simulink model "LEGO_PendulumOnCart"  (R2013b)
settings: Solver=ode3  SolverMode=SingleTasking  StartTime=0.0  StopTime=13  FixedStep=ts1  RelTol=1e-3
PostLoadFcn:
  | LEGO_PendulumOnCart_plant;
  | LEGO_PendulumOnCart_controller;
  | LEGO_PendulumOnCart_simulation;
InitFcn:
  | LEGO_PendulumOnCart_plant;
  | LEGO_PendulumOnCart_controller;
  | LEGO_PendulumOnCart_simulation;
values from neighbouring files (symbols this model uses):
  a_b = 0.8    [LEGO_PendulumOnCart_controller.m]    (also in matlab.mat)
  a_d = 0.8    [LEGO_PendulumOnCart_controller.m]    (also in matlab.mat)
  ANGLE_OFFSET = 93    [LEGO_PendulumOnCart_controller.m]    (also in matlab.mat = 48)
  cm2phi = 2    [LEGO_PendulumOnCart_controller.m]    (also in matlab.mat = 1)
  k_cp = 0.5    [matlab.mat]
  k_gv = w_n^2/(212.4*k_v)    (= 1.61490625454)    [LEGO_PendulumOnCart_controller.m]    (also in matlab.mat)
  k_v = (w_n^2-2826)/212.4    (= 21.6375823917)    [LEGO_PendulumOnCart_controller.m]    (also in matlab.mat)
  k_z = -2*w_n1    [LEGO_PendulumOnCart_controller.m]    (also in matlab.mat = -15.1928775883)
  l = 0.17    [LEGO_PendulumOnCart_controller.m]    (also in LEGO_PendulumOnCart_plant.m; matlab.mat)
  R = 0.025    [LEGO_PendulumOnCart_plant.m]    (also in matlab.mat)
  ts1 = 0.004    [LEGO Servo Motor experiments.mat]    (also in LEGO_PendulumOnCart_controller.m; matlab.mat)
undefined symbols (not defined in the file or in its folder): Normalized, sigbuilder_block
libraries: legonxtlib x10, simulink x3
CloseFcn:
  | LEGO_PendulumOnCart_closemodel;
Description:
  | This is an Implementation of Pendulum on a cart system using LEGO Mindstorms NXT Kit.
settings Model: ExtModeTrigDuration=2  Creator=Alphonso Monk  LastModifiedBy=Alphonso Monk
settings OptimizationCC: OptimizeModelRefInitCode=on  LifeSpan=1
settings DebuggingCC: SolverPrmCheckMsg=none
settings HardwareCC: ProdLargestAtomicInteger=Long  ProdLargestAtomicFloat=Float  ProdEndianess=LittleEndian  ProdHWDeviceType=ARM Compatible->ARM 7
settings SFSimCC: SimParseCustomCode=off
settings RTWCC: SystemTargetFile=realtime.tlc  GenerateMakefile=off  TemplateMakefile=realtime.tmf  Description=Run on Target Hardware  RTWVerbose=off  ProcessScript=realtime_make_rtw_hook
settings CodeAppCC: InternalIdentifier=Classic
settings STFCustomTargetCC: TargetLibSuffix=.a  GenerateSampleERTMain=on  ERTCustomFileBanners=on  SupportNonInlinedSFcns=off  SupportVariableSizeSignals=on  MATLABClassNameForMDSCustomization=Simulink.SoftwareTarget.ERTCustomization  GRTInterface=off  SystemTargetFile=realtime.tlc
settings ERTTargetCC: CodeReplacementLibrary=ANSI_C  GenerateSampleERTMain=on  ParMdlRefBuildCompliant=off  CompOptLevelCompliant=off  ConcurrentExecutionCompliant=off  CombineOutputUpdateFcns=off  ERTFirstTimeCompliant=off  SupportContinuousTime=on  SupportVariableSizeSignals=on  ModelStepFunctionPrototypeControlCompliant=off  CPPClassGenCompliant=off  ExtMode=on  ExtModeTransport=2  ExtModeMexFile=ext_serial_win32_comm_no_acks_rtt  ExtModeMexArgs=0 3 9600 30  InlinedParameterPlacement=NonHierarchical  ERTSrcFileBannerTemplate=realtime_code_template.cgt  ERTHdrFileBannerTemplate=realtime_code_template.cgt  ERTDataSrcFileTemplate=realtime_code_template.cgt  ERTDataHdrFileTemplate=realtime_code_template.cgt  ERTCustomFileTemplate=realtime_file_process.tlc

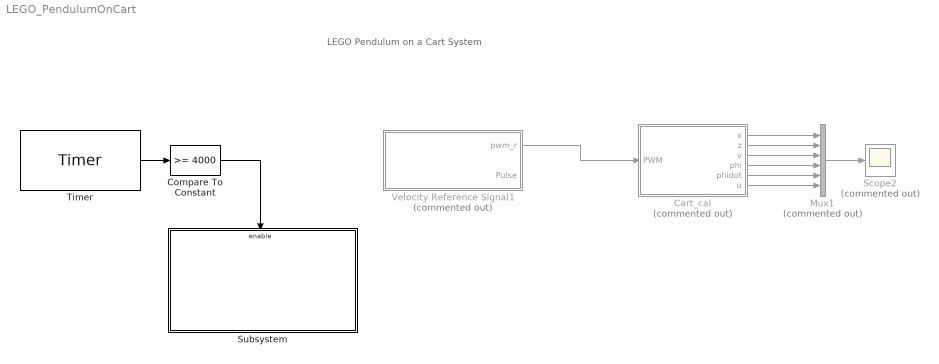
== system LEGO_PendulumOnCart ==
  note: LEGO Pendulum on a Cart System
  Cart_cal : Subsystem  Commented=on
  Compare To Constant : simulink/Logic and Bit Operations/Compare To Constant  relop=>=  const=4000  OutDataTypeStr=boolean
  Mux1 : Mux  Commented=on  Inputs=6
  Scope2 : Scope  Commented=on
      settings: YMin=-25  YMax=50  SaveName=PendulumOnCart_scope2
  Subsystem : Subsystem
  Timer : legonxtlib/Timer  sampleTime=0.1
  Velocity Reference Signal1 : Subsystem  Tag=STV Subsys  Commented=on  LoadFcn=sigbuilder_block('load');  StartFcn=sigbuilder_block('start');  StopFcn=sigbuilder_block('stop');  ClipboardFcn=sigbuilder_block('clipboard');  mask(Sigbuilder block){}
      mask help: Simulink:masks:SigbuilderBlock_MD
      mask init:
      | if ~strcmp(get_param(bdroot(gcbh),'SimulationStatus'),'stopped') tuvar = sigbuilder_block('maskInit'); end
      settings: CopyFcn=sigbuilder_block('copy');  DeleteFcn=sigbuilder_block('delete');  ModelCloseFcn=sigbuilder_block('modelClose');  PreSaveFcn=sigbuilder_block('preSave');  PauseFcn=sigbuilder_block('pause');  ContinueFcn=sigbuilder_block('continue');  NameChangeFcn=sigbuilder_block('namechange');  OpenFcn=sigbuilder_block('open',[437.25 118.5 550.5 394.5 ]);  CloseFcn=sigbuilder_block('close');
      mask Display: plot(0, 0, 100, 100,[2, 2, 32, 32, 2], [68, 8, 8, 68, 68],[32, 2], [38, 38], [32, 19, 2],[53, 60, 44], [32, 17, 17, 2],[16, 16, 31, 31]);txt = getActiveGroup(gcbh);text(2, 100, txt,'verticalAlignment', 'top');
  wires:
  Cart_cal/4(phi) -> Mux1/4
  Mux1/1 -> Scope2/1
  Velocity Reference Signal1/1(pwm_r) -> Cart_cal/1(PWM)
  Cart_cal/1(x) -> Mux1/1
  Cart_cal/2(z) -> Mux1/2
  Cart_cal/3(v) -> Mux1/3
  Cart_cal/5(phidot) -> Mux1/5
  Cart_cal/6(u) -> Mux1/6
  Compare To Constant/1 -> Subsystem/Enable
  Timer/1 -> Compare To Constant/1

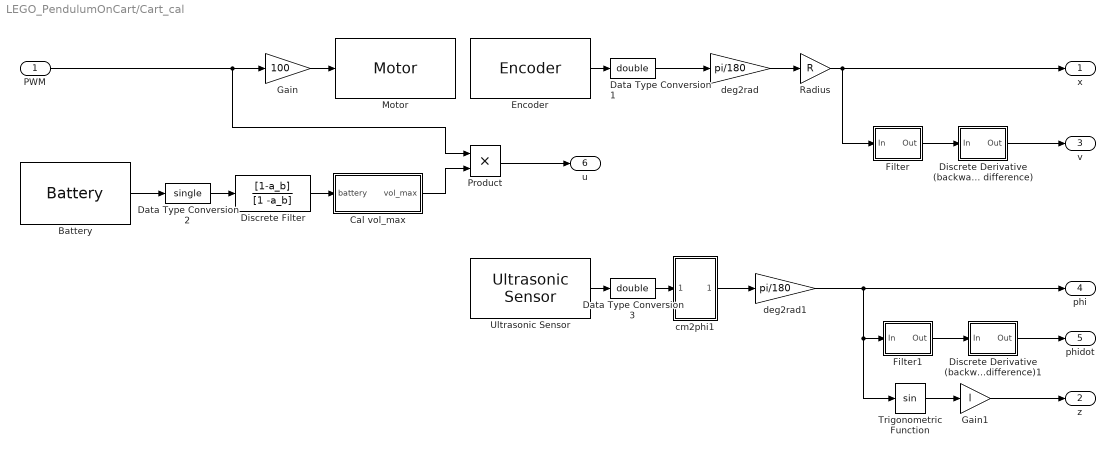
== system LEGO_PendulumOnCart/Cart_cal ==
  PWM : Inport
  Battery : legonxtlib/Battery  sampleTime=ts1
  Cal vol_max : Subsystem
  Data Type Conversion1 : DataTypeConversion  OutDataTypeStr=double  RndMeth=Simplest
  Data Type Conversion2 : DataTypeConversion  OutDataTypeStr=single  RndMeth=Simplest
  Data Type Conversion3 : DataTypeConversion  OutDataTypeStr=double  RndMeth=Simplest
  Discrete Derivative (backward difference) : Subsystem
  Discrete Derivative (backward difference)1 : Subsystem
  Discrete Filter : DiscreteFilter  Numerator=[1-a_b]  Denominator=[1 -a_b]
  Encoder : legonxtlib/Encoder  portNumber=B  opMode=No reset  sampleTime=ts1
  Filter : Subsystem
  Filter1 : Subsystem
  Gain : Gain  Gain=100
  Gain1 : Gain  Gain=l
  Motor : legonxtlib/Motor  sportNumber=B  sstopAction=Brake
  Product : Product
  Radius : Gain  Gain=R
  Trigonometric Function : Trigonometry
  Ultrasonic Sensor : legonxtlib/Ultrasonic Sensor  PortNumber=4  sampleTime=ts1
  cm2phi1 : Subsystem
  deg2rad : Gain  Gain=pi/180
  deg2rad1 : Gain  Gain=pi/180
  x : Outport
  z : Outport  Port=2
  v : Outport  Port=3
  phi : Outport  Port=4
  phidot : Outport  Port=5
  u : Outport  Port=6
  wires:
  Gain1/1 -> z/1
  Trigonometric Function/1 -> Gain1/1
  cm2phi1/1(phi) -> deg2rad1/1
  Discrete Derivative (backward difference)1/1(Out) -> phidot/1
  Ultrasonic Sensor/1 -> Data Type Conversion3/1
  Filter1/1(Out) -> Discrete Derivative (backward difference)1/1(In)
  Data Type Conversion3/1 -> cm2phi1/1(cm)
  Discrete Derivative (backward difference)/1(Out) -> v/1
  Filter/1(Out) -> Discrete Derivative (backward difference)/1(In)
  Data Type Conversion1/1 -> deg2rad/1
  Battery/1 -> Data Type Conversion2/1
  Data Type Conversion2/1 -> Discrete Filter/1
  Discrete Filter/1 -> Cal vol_max/1(battery)
  PWM/1 -> Gain/1, Product/1
  Cal vol_max/1(vol_max) -> Product/2
  Radius/1 -> x/1, Filter/1(In)
  Encoder/1 -> Data Type Conversion1/1
  Gain/1 -> Motor/1
  Product/1 -> u/1
  deg2rad/1 -> Radius/1
  deg2rad1/1 -> phi/1, Filter1/1(In), Trigonometric Function/1

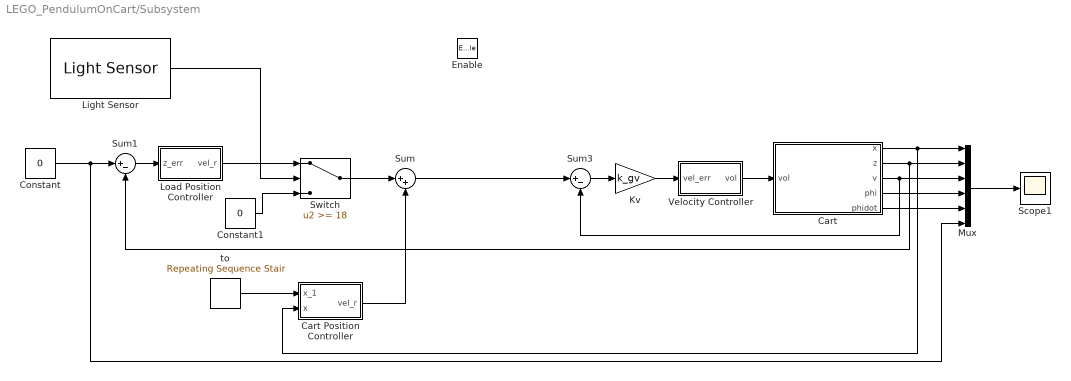
== system LEGO_PendulumOnCart/Subsystem ==
  Enable : EnablePort
  Cart : Subsystem
  Cart Position Controller : Subsystem
  Constant : Constant  Value=0
  Constant1 : Constant  Value=0
  Kv : Gain  Gain=k_gv
  Light Sensor : legonxtlib/Light Sensor  portNumber=1  outputMode=Normalized (0 -100)  lightOn=off  sampleTime=0.1
  Load Position Controller : Subsystem
  Mux : Mux  Inputs=6
  Scope1 : Scope
      settings: TimeRange=50  YMin=1026  YMax=1134  SaveName=PendulumOnCart_scope1
  Sum : Sum  Inputs=|++
  Sum1 : Sum  Inputs=|+-
  Sum3 : Sum  Inputs=|+-
  Switch : Switch  Threshold=18
  Velocity Controller : Subsystem
  to : simulink/Sources/Repeating Sequence Stair  OutValues=[0 0 0 1 1 1 1 1 0 0].'  tsamp=2  OutMin=[]  OutMax=[]  OutDataTypeStr=double  OutputDataTypeScalingMode=double  OutDataType=fixdt(0,8)  ConRadixGroup=Best Precision: Vector-wise  OutScaling=2^-12
  wires:
  Velocity Controller/1(vol) -> Cart/1(vol)
  Cart/3(v) -> Mux/3, Sum3/2
  Cart/1(x) -> Cart Position Controller/2(x), Mux/1
  Sum1/1 -> Load Position Controller/1(z_err)
  Constant/1 -> Sum1/1, Mux/6
  Cart/2(z) -> Mux/2, Sum1/2
  Cart/4(phi) -> Mux/4
  Cart/5(phidot) -> Mux/5
  Mux/1 -> Scope1/1
  Kv/1 -> Velocity Controller/1(vel_err)
  Sum/1 -> Sum3/1
  Cart Position Controller/1(vel_r) -> Sum/2
  Switch/1 -> Sum/1
  Load Position Controller/1(vel_r) -> Switch/1
  Light Sensor/1 -> Switch/2
  Constant1/1 -> Switch/3
  to/1 -> Cart Position Controller/1(x_1)
  Sum3/1 -> Kv/1

== system LEGO_PendulumOnCart/Velocity Reference Signal1 ==
  Demux : Demux  Tag=STV Demux  Outputs=2
  FromWs : FromWorkspace  Tag=STV FromWs  VariableName=tuvar  SampleTime=0
      SigBuilderData=|
      | common.afterFinalStr = 'Extrapolate'
      | common.sampleTime = 0
      | dataSet.timeRange = [0 100]
      | dataSet.name = 'Velocity Control'
      | sbobj.Groups.Name = 'Velocity Control'
      | sbobj.Groups.Signals(1).Name = 'pwm_r'
      | sbobj.Groups.Signals(1).XData = [0 4 4 8 8 14 14 16 16 20 20 22 22 24 24 28 28 36 36 38 38 48 48 50 50 52 52 54 54 56 56 64 64 68 68 70 70 72 72 78 78 82 82 88 88 94 94 96 96 100]
      | sbobj.Groups.Signals(1).YData = [1 1 -1 -1 1 1 -1 -1 1 1 -1 -1 1 1 -1 -1 1 1 -1 -1 1 1 -1 -1 1 1 -1 -1 1 1 -1 -1 1 1 -1 -1 1 1 -1 -1 1 1 -1 -1 1 1 -1 -1 1 1]
      | sbobj.Groups.Signals(2).Name = 'Pulse'
      | sbobj.Groups.Signals(2).XData = [0 5 5 10 10 100]
      | sbobj.Groups.Signals(2).YData = [0 0 1 1 0 0]
      | sbobj.Groups.TimeRange = [0 100]
  pwm_r : Outport  Tag=STV Outport
  Pulse : Outport  Tag=STV Outport  Port=2
  wires:
  FromWs/1 -> Demux/1
  Demux/1 -> pwm_r/1
  Demux/2 -> Pulse/1

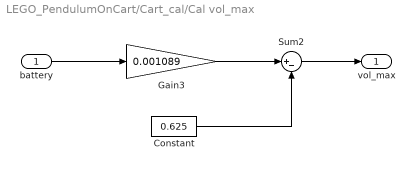
== system LEGO_PendulumOnCart/Cart_cal/Cal vol_max ==
  battery : Inport
  Constant : Constant  Value=0.625  OutDataTypeStr=single
      settings: AttributesFormatString=DataType = %<OutDataTypeStr>
  Gain3 : Gain  Gain=0.001089  OutDataTypeStr=Inherit: Same as input  ParamDataTypeStr=Inherit: Same as input
  Sum2 : Sum  Inputs=|+-  OutDataTypeStr=Inherit: Same as first input
  vol_max : Outport
  wires:
  battery/1 -> Gain3/1
  Constant/1 -> Sum2/2
  Sum2/1 -> vol_max/1
  Gain3/1 -> Sum2/1

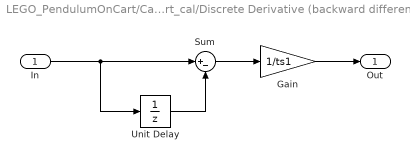
== system LEGO_PendulumOnCart/Cart_cal/Discrete Derivative (backward difference) ==
  In : Inport
  Gain : Gain  Gain=1/ts1  OutDataTypeStr=Inherit: Same as input  ParamDataTypeStr=Inherit: Same as input
  Sum : Sum  Inputs=|+-  OutDataTypeStr=Inherit: Same as first input
  Unit Delay : UnitDelay  SampleTime=-1
  Out : Outport
  wires:
  Gain/1 -> Out/1
  In/1 -> Sum/1, Unit Delay/1
  Unit Delay/1 -> Sum/2
  Sum/1 -> Gain/1

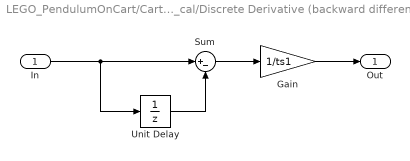
== system LEGO_PendulumOnCart/Cart_cal/Discrete Derivative (backward difference)1 ==
  In : Inport
  Gain : Gain  Gain=1/ts1  OutDataTypeStr=Inherit: Same as input  ParamDataTypeStr=Inherit: Same as input
  Sum : Sum  Inputs=|+-  OutDataTypeStr=Inherit: Same as first input
  Unit Delay : UnitDelay  SampleTime=-1
  Out : Outport
  wires:
  Sum/1 -> Gain/1
  Unit Delay/1 -> Sum/2
  In/1 -> Unit Delay/1, Sum/1
  Gain/1 -> Out/1

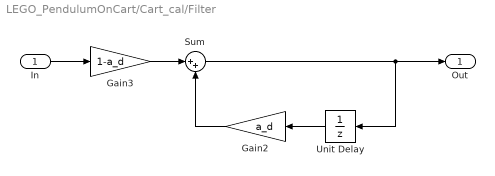
== system LEGO_PendulumOnCart/Cart_cal/Filter ==
  In : Inport
  Gain2 : Gain  Gain=a_d  OutDataTypeStr=Inherit: Same as input  ParamDataTypeStr=Inherit: Same as input
  Gain3 : Gain  Gain=1-a_d  OutDataTypeStr=Inherit: Same as input  ParamDataTypeStr=Inherit: Same as input
  Sum : Sum  Inputs=|++  OutDataTypeStr=Inherit: Same as first input
  Unit Delay : UnitDelay  SampleTime=-1
  Out : Outport
  wires:
  In/1 -> Gain3/1
  Gain3/1 -> Sum/1
  Gain2/1 -> Sum/2
  Unit Delay/1 -> Gain2/1
  Sum/1 -> Out/1, Unit Delay/1

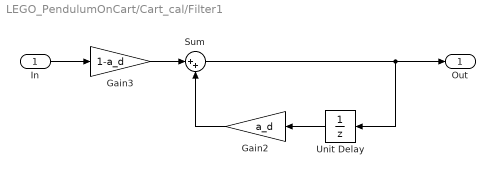
== system LEGO_PendulumOnCart/Cart_cal/Filter1 ==
  In : Inport
  Gain2 : Gain  Gain=a_d  OutDataTypeStr=Inherit: Same as input  ParamDataTypeStr=Inherit: Same as input
  Gain3 : Gain  Gain=1-a_d  OutDataTypeStr=Inherit: Same as input  ParamDataTypeStr=Inherit: Same as input
  Sum : Sum  Inputs=|++  OutDataTypeStr=Inherit: Same as first input
  Unit Delay : UnitDelay  SampleTime=-1
  Out : Outport
  wires:
  Sum/1 -> Unit Delay/1, Out/1
  Unit Delay/1 -> Gain2/1
  Gain2/1 -> Sum/2
  Gain3/1 -> Sum/1
  In/1 -> Gain3/1

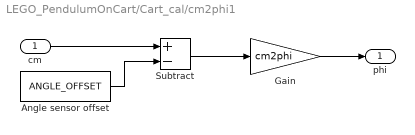
== system LEGO_PendulumOnCart/Cart_cal/cm2phi1 ==
  cm : Inport
  Angle sensor offset : Constant  Value=ANGLE_OFFSET
  Gain : Gain  Gain=cm2phi
  Subtract : Sum  Inputs=+-
  phi : Outport
  wires:
  Gain/1 -> phi/1
  Subtract/1 -> Gain/1
  Angle sensor offset/1 -> Subtract/2
  cm/1 -> Subtract/1

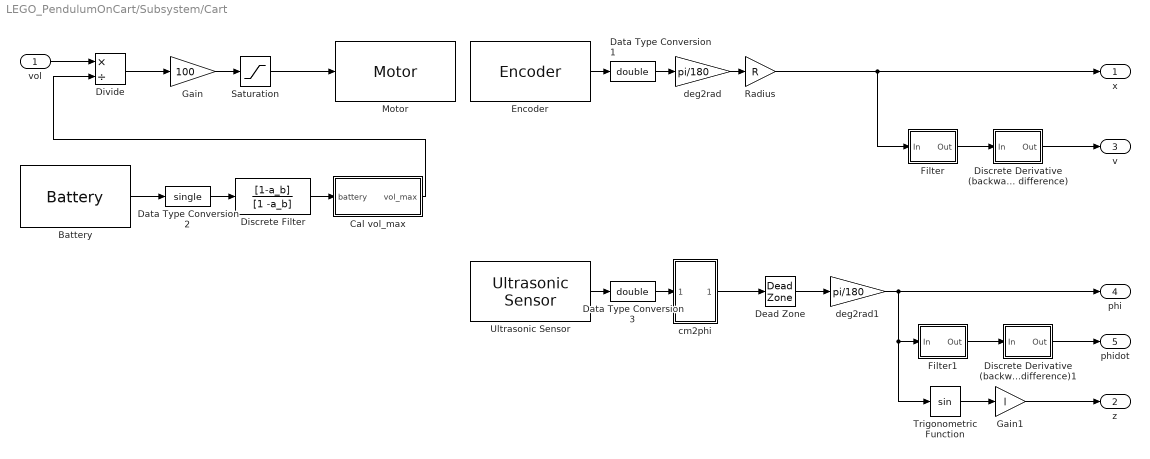
== system LEGO_PendulumOnCart/Subsystem/Cart ==
  vol : Inport
  Battery : legonxtlib/Battery  sampleTime=ts1
  Cal vol_max : Subsystem
  Data Type Conversion1 : DataTypeConversion  OutDataTypeStr=double  RndMeth=Simplest
  Data Type Conversion2 : DataTypeConversion  OutDataTypeStr=single  RndMeth=Simplest
  Data Type Conversion3 : DataTypeConversion  OutDataTypeStr=double  RndMeth=Simplest
  Dead Zone : DeadZone  LowerValue=-2  UpperValue=2  SaturateOnIntegerOverflow=on
  Discrete Derivative (backward difference) : Subsystem
  Discrete Derivative (backward difference)1 : Subsystem
  Discrete Filter : DiscreteFilter  Numerator=[1-a_b]  Denominator=[1 -a_b]
  Divide : Product  Inputs=*/
  Encoder : legonxtlib/Encoder  portNumber=B  opMode=No reset  sampleTime=ts1
  Filter : Subsystem
  Filter1 : Subsystem
  Gain : Gain  Gain=100
  Gain1 : Gain  Gain=l
  Motor : legonxtlib/Motor  sportNumber=B  sstopAction=Brake
  Radius : Gain  Gain=R
  Saturation : Saturate  UpperLimit=100  LowerLimit=-100
  Trigonometric Function : Trigonometry  OutputSignalType=real
  Ultrasonic Sensor : legonxtlib/Ultrasonic Sensor  PortNumber=4  sampleTime=ts1
  cm2phi : Subsystem
  deg2rad : Gain  Gain=pi/180
  deg2rad1 : Gain  Gain=pi/180
  x : Outport
  z : Outport  Port=2
  v : Outport  Port=3
  phi : Outport  Port=4
  phidot : Outport  Port=5
  wires:
  Encoder/1 -> Data Type Conversion1/1
  Radius/1 -> Filter/1(In), x/1
  Saturation/1 -> Motor/1
  Divide/1 -> Gain/1
  Cal vol_max/1(vol_max) -> Divide/2
  vol/1 -> Divide/1
  Discrete Filter/1 -> Cal vol_max/1(battery)
  Data Type Conversion2/1 -> Discrete Filter/1
  Battery/1 -> Data Type Conversion2/1
  Gain/1 -> Saturation/1
  Data Type Conversion1/1 -> deg2rad/1
  Filter/1(Out) -> Discrete Derivative (backward difference)/1(In)
  Discrete Derivative (backward difference)/1(Out) -> v/1
  Data Type Conversion3/1 -> cm2phi/1(cm)
  Filter1/1(Out) -> Discrete Derivative (backward difference)1/1(In)
  Ultrasonic Sensor/1 -> Data Type Conversion3/1
  Discrete Derivative (backward difference)1/1(Out) -> phidot/1
  cm2phi/1(phi) -> Dead Zone/1
  Trigonometric Function/1 -> Gain1/1
  Gain1/1 -> z/1
  deg2rad/1 -> Radius/1
  deg2rad1/1 -> Trigonometric Function/1, Filter1/1(In), phi/1
  Dead Zone/1 -> deg2rad1/1

== system LEGO_PendulumOnCart/Subsystem/Cart Position Controller ==
  x_1 : Inport
  x : Inport  Port=2
  Discrete PID Controller : simulink/Continuous/PID Controller  Controller=PID  TimeDomain=Discrete-time  SampleTime=ts1  IntegratorMethod=Forward Euler  FilterMethod=Forward Euler  Form=Parallel  P=k_cp  I=0  D=0  N=100  InitialConditionSource=internal  InitialConditionForIntegrator=0  InitialConditionForFilter=0  ExternalReset=none  LimitOutput=on  UpperSaturationLimit=0.5  LowerSaturationLimit=-0.5  LinearizeAsGain=off  AntiWindupMode=none  Kb=1  TrackingMode=off  Kt=1  PParamMin=[]  PParamMax=[]  IParamMin=[]  IParamMax=[]  DParamMin=[]  DParamMax=[]  NParamMin=[]  NParamMax=[]  KbParamMin=[]  KbParamMax=[]  KtParamMin=[]  KtParamMax=[]  POutMin=[]  POutMax=[]  IOutMin=[]  IOutMax=[]  DOutMin=[]  DOutMax=[]  NOutMin=[]  NOutMax=[]  KbOutMin=[]  KbOutMax=[]  KtOutMin=[]  KtOutMax=[]  IntegratorOutMin=[]  IntegratorOutMax=[]  FilterOutMin=[]  FilterOutMax=[]  SumOutMin=[]  SumOutMax=[]  SumI1OutMin=[]  SumI1OutMax=[]  SumI2OutMin=[]  SumI2OutMax=[]  SumI3OutMin=[]  SumI3OutMax=[]  SumDOutMin=[]  SumDOutMax=[]  SaturationOutMin=[]  SaturationOutMax=[]  IntegratorContinuousStateAttributes=''  IntegratorStateMustResolveToSignalObject=off  IntegratorRTWStateStorageClass=Auto  FilterContinuousStateAttributes=''  FilterStateMustResolveToSignalObject=off  FilterRTWStateStorageClass=Auto
  Sum2 : Sum  Inputs=|+-
  vel_r : Outport
  wires:
  x_1/1 -> Sum2/1
  Sum2/1 -> Discrete PID Controller/1
  x/1 -> Sum2/2
  Discrete PID Controller/1 -> vel_r/1

== system LEGO_PendulumOnCart/Subsystem/Load Position Controller ==
  z_err : Inport
  Kz : Gain  Gain=k_z
  vel_r : Outport
  wires:
  z_err/1 -> Kz/1
  Kz/1 -> vel_r/1

== system LEGO_PendulumOnCart/Subsystem/Velocity Controller ==
  vel_err : Inport
  Kv : Gain  Gain=k_v
  vol : Outport
  wires:
  Kv/1 -> vol/1
  vel_err/1 -> Kv/1

== system LEGO_PendulumOnCart/Subsystem/Cart/Cal vol_max ==
  battery : Inport
  Constant : Constant  Value=0.625  OutDataTypeStr=single
      settings: AttributesFormatString=DataType = %<OutDataTypeStr>
  Gain3 : Gain  Gain=0.001089  OutDataTypeStr=Inherit: Same as input  ParamDataTypeStr=Inherit: Same as input
  Sum2 : Sum  Inputs=|+-  OutDataTypeStr=Inherit: Same as first input
  vol_max : Outport
  wires:
  Gain3/1 -> Sum2/1
  Sum2/1 -> vol_max/1
  Constant/1 -> Sum2/2
  battery/1 -> Gain3/1

== system LEGO_PendulumOnCart/Subsystem/Cart/Discrete Derivative (backward difference) ==
  In : Inport
  Gain : Gain  Gain=1/ts1  OutDataTypeStr=Inherit: Same as input  ParamDataTypeStr=Inherit: Same as input
  Sum : Sum  Inputs=|+-  OutDataTypeStr=Inherit: Same as first input
  Unit Delay : UnitDelay  SampleTime=-1
  Out : Outport
  wires:
  Sum/1 -> Gain/1
  Unit Delay/1 -> Sum/2
  In/1 -> Unit Delay/1, Sum/1
  Gain/1 -> Out/1

== system LEGO_PendulumOnCart/Subsystem/Cart/Discrete Derivative (backward difference)1 ==
  In : Inport
  Gain : Gain  Gain=1/ts1  OutDataTypeStr=Inherit: Same as input  ParamDataTypeStr=Inherit: Same as input
  Sum : Sum  Inputs=|+-  OutDataTypeStr=Inherit: Same as first input
  Unit Delay : UnitDelay  SampleTime=-1
  Out : Outport
  wires:
  Gain/1 -> Out/1
  In/1 -> Sum/1, Unit Delay/1
  Unit Delay/1 -> Sum/2
  Sum/1 -> Gain/1

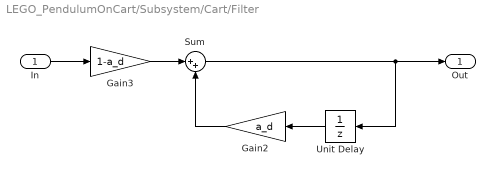
== system LEGO_PendulumOnCart/Subsystem/Cart/Filter ==
  In : Inport
  Gain2 : Gain  Gain=a_d  OutDataTypeStr=Inherit: Same as input  ParamDataTypeStr=Inherit: Same as input
  Gain3 : Gain  Gain=1-a_d  OutDataTypeStr=Inherit: Same as input  ParamDataTypeStr=Inherit: Same as input
  Sum : Sum  Inputs=|++  OutDataTypeStr=Inherit: Same as first input
  Unit Delay : UnitDelay  SampleTime=-1
  Out : Outport
  wires:
  Sum/1 -> Unit Delay/1, Out/1
  Unit Delay/1 -> Gain2/1
  Gain2/1 -> Sum/2
  Gain3/1 -> Sum/1
  In/1 -> Gain3/1

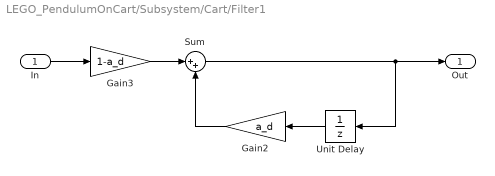
== system LEGO_PendulumOnCart/Subsystem/Cart/Filter1 ==
  In : Inport
  Gain2 : Gain  Gain=a_d  OutDataTypeStr=Inherit: Same as input  ParamDataTypeStr=Inherit: Same as input
  Gain3 : Gain  Gain=1-a_d  OutDataTypeStr=Inherit: Same as input  ParamDataTypeStr=Inherit: Same as input
  Sum : Sum  Inputs=|++  OutDataTypeStr=Inherit: Same as first input
  Unit Delay : UnitDelay  SampleTime=-1
  Out : Outport
  wires:
  In/1 -> Gain3/1
  Gain3/1 -> Sum/1
  Gain2/1 -> Sum/2
  Unit Delay/1 -> Gain2/1
  Sum/1 -> Out/1, Unit Delay/1

== system LEGO_PendulumOnCart/Subsystem/Cart/cm2phi ==
  cm : Inport
  Angle sensor offset : Constant  Value=ANGLE_OFFSET
  Gain : Gain  Gain=cm2phi
  Subtract : Sum  Inputs=+-
  phi : Outport
  wires:
  Gain/1 -> phi/1
  Subtract/1 -> Gain/1
  Angle sensor offset/1 -> Subtract/2
  cm/1 -> Subtract/1
